simulink model "Privod"  (R2023a)
settings: Solver=ode15s  StartTime=0.0  StopTime=4  RelTol=1e-3
undefined symbols (not defined in the file): a, ak0, ak1, ap0, ap1, bk0, bk1, bp0, bp1, c, F1, F2, G, G1, G2, i, J, k1, k2, Kc, Ki, kip, Kk, km, kpd, kpid, kv, T
settings Model: Creator=manui  LastModifiedBy=manui

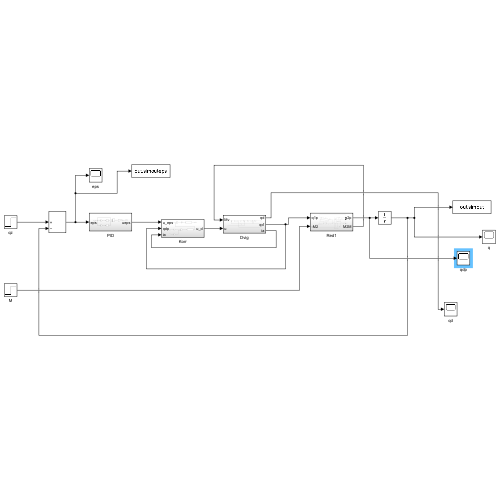
[thumbnail: Simulink's stored preview of the top-level diagram]
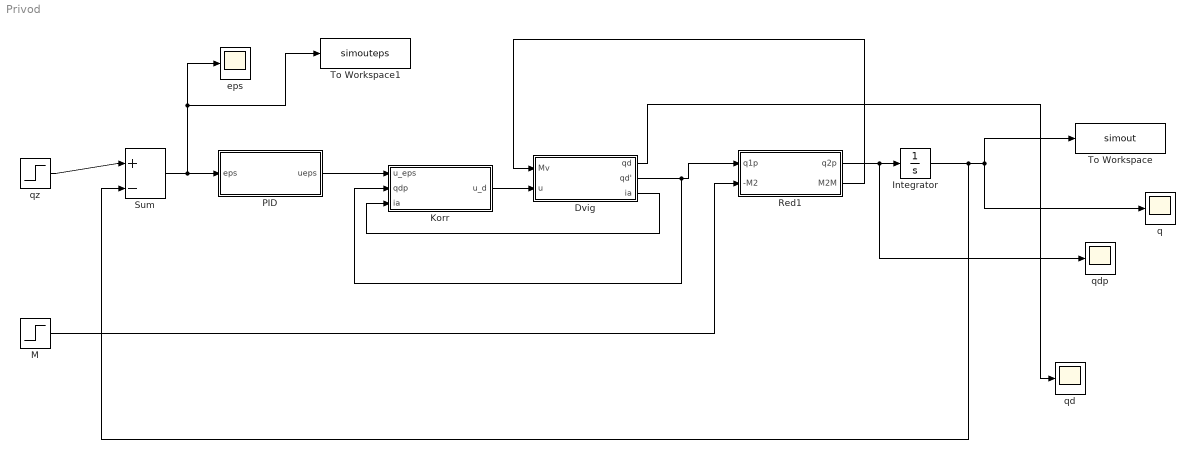
== system Privod ==
  Dvig : Subsystem
  Integrator : Integrator
  Korr : Subsystem
  M : Step  Time=0  After=0  SampleTime=0
  PID : Subsystem
  Red1 : Subsystem
  Sum : Sum  Inputs=|+-
  To Workspace : ToWorkspace  VariableName=simout  SaveFormat=Timeseries  SampleTime=-1
  To Workspace1 : ToWorkspace  VariableName=simouteps  SaveFormat=Timeseries  SampleTime=-1
  eps : Scope
  q : Scope
  qd : Scope
  qdp : Scope
  qz : Step  Time=0  After=0.1  SampleTime=0
  wires:
  qz/1 -> Sum/1
  Sum/1 -> To Workspace1/1, eps/1, PID/1(eps)
  PID/1(ueps) -> Korr/1(u_eps)
  Korr/1(u_d) -> Dvig/2(u)
  Dvig/3(ia) -> Korr/3(ia)
  Dvig/2(qd') -> Korr/2(qdp), Red1/1(q1p)
  M/1 -> Red1/2(-M2)
  Dvig/1(qd) -> qd/1
  Red1/2(M2M) -> Dvig/1(Mv)
  Red1/1(q2p) -> qdp/1, Integrator/1
  Integrator/1 -> Sum/2, To Workspace/1, q/1

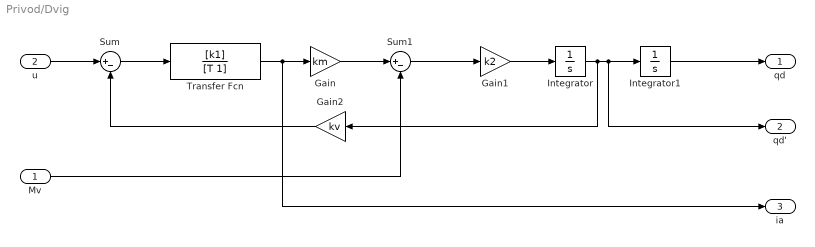
== system Privod/Dvig ==
  Mv : Inport
  u : Inport  Port=2
  Gain : Gain  Gain=km
  Gain1 : Gain  Gain=k2
  Gain2 : Gain  Gain=kv
  Integrator : Integrator
  Integrator1 : Integrator
  Sum : Sum  Inputs=|+-
  Sum1 : Sum  Inputs=|+-
  Transfer Fcn : TransferFcn  Numerator=[k1]  Denominator=[T 1]
  qd : Outport
  qd' : Outport  Port=2
  ia : Outport  Port=3
  wires:
  u/1 -> Sum/1
  Sum/1 -> Transfer Fcn/1
  Transfer Fcn/1 -> ia/1, Gain/1
  Gain/1 -> Sum1/1
  Mv/1 -> Sum1/2
  Sum1/1 -> Gain1/1
  Gain1/1 -> Integrator/1
  Integrator/1 -> Gain2/1, qd'/1, Integrator1/1
  Integrator1/1 -> qd/1
  Gain2/1 -> Sum/2

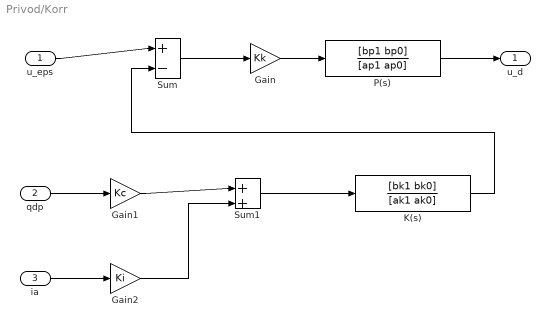
== system Privod/Korr ==
  u_eps : Inport
  qdp : Inport  Port=2
  ia : Inport  Port=3
  Gain : Gain  Gain=Kk
  Gain1 : Gain  Gain=Kc
  Gain2 : Gain  Gain=Ki
  K(s) : TransferFcn  Numerator=[bk1 bk0]  Denominator=[ak1 ak0]
  P(s) : TransferFcn  Numerator=[bp1 bp0]  Denominator=[ap1 ap0]
  Sum : Sum  Inputs=|+-
  Sum1 : Sum  Inputs=|++
  u_d : Outport
  wires:
  Sum/1 -> Gain/1
  u_eps/1 -> Sum/1
  Gain/1 -> P(s)/1
  P(s)/1 -> u_d/1
  qdp/1 -> Gain1/1
  Gain1/1 -> Sum1/1
  Sum1/1 -> K(s)/1
  Gain2/1 -> Sum1/2
  ia/1 -> Gain2/1
  K(s)/1 -> Sum/2

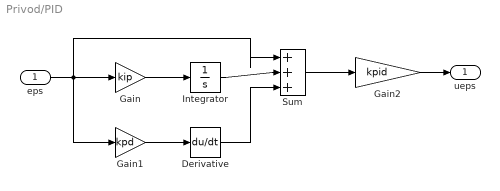
== system Privod/PID ==
  eps : Inport
  Derivative : Derivative
  Gain : Gain  Gain=kip
  Gain1 : Gain  Gain=kpd
  Gain2 : Gain  Gain=kpid
  Integrator : Integrator
  Sum : Sum  Inputs=|+++
  ueps : Outport
  wires:
  eps/1 -> Gain1/1, Sum/1, Gain/1
  Gain/1 -> Integrator/1
  Integrator/1 -> Sum/2
  Gain1/1 -> Derivative/1
  Derivative/1 -> Sum/3
  Sum/1 -> Gain2/1
  Gain2/1 -> ueps/1

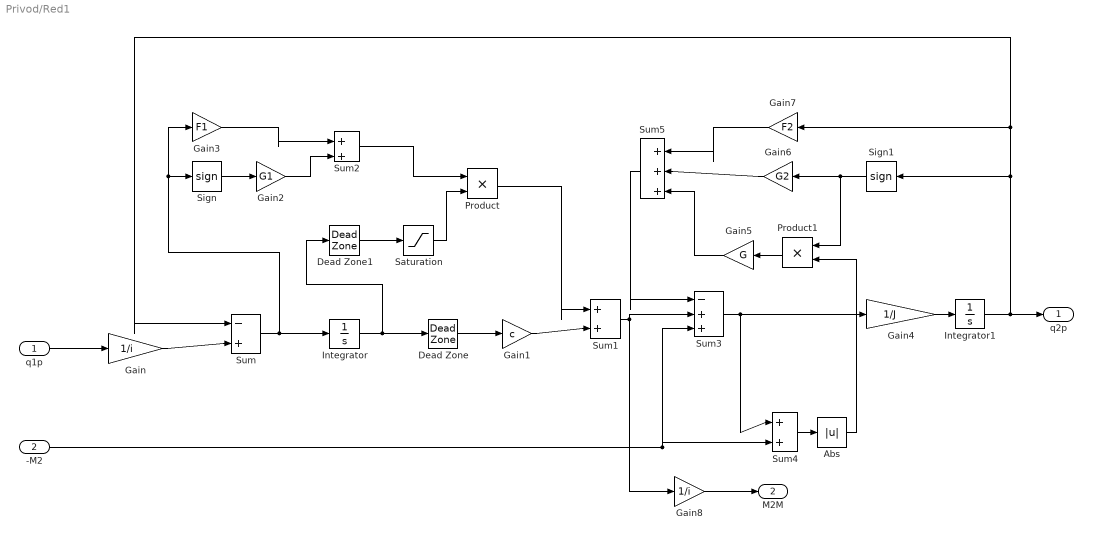
== system Privod/Red1 ==
  q1p : Inport
  -M2 : Inport  Port=2
  Abs : Abs  SaturateOnIntegerOverflow=off
  Dead Zone : DeadZone  LowerValue=-a  UpperValue=a
  Dead Zone1 : DeadZone  LowerValue=-a  UpperValue=a
  Gain : Gain  Gain=1/i
  Gain1 : Gain  Gain=c
  Gain2 : Gain  Gain=G1
  Gain3 : Gain  Gain=F1
  Gain4 : Gain  Gain=1/J
  Gain5 : Gain  Gain=G
  Gain6 : Gain  Gain=G2
  Gain7 : Gain  Gain=F2
  Gain8 : Gain  Gain=1/i
  Integrator : Integrator
  Integrator1 : Integrator
  Product : Product
  Product1 : Product
  Saturation : Saturate  UpperLimit=a  LowerLimit=-a
  Sign : Signum
  Sign1 : Signum
  Sum : Sum  Inputs=|-+
  Sum1 : Sum  Inputs=|++
  Sum2 : Sum  Inputs=|++
  Sum3 : Sum  Inputs=|-++
  Sum4 : Sum  Inputs=|++
  Sum5 : Sum  Inputs=|+++
  q2p : Outport
  M2M : Outport  Port=2
  wires:
  q1p/1 -> Gain/1
  Gain/1 -> Sum/2
  Sum/1 -> Sign/1, Gain3/1, Integrator/1
  Integrator/1 -> Dead Zone1/1, Dead Zone/1
  Dead Zone/1 -> Gain1/1
  Gain1/1 -> Sum1/2
  Product/1 -> Sum1/1
  Saturation/1 -> Product/2
  Dead Zone1/1 -> Saturation/1
  Gain2/1 -> Sum2/2
  Sum2/1 -> Product/1
  Gain3/1 -> Sum2/1
  Sign/1 -> Gain2/1
  Sum1/1 -> Gain8/1, Sum3/2
  -M2/1 -> Sum3/3, Sum4/2
  Gain4/1 -> Integrator1/1
  Integrator1/1 -> Sum/1, Gain7/1, Sign1/1, q2p/1
  Sum3/1 -> Sum4/1, Gain4/1
  Sum4/1 -> Abs/1
  Abs/1 -> Product1/2
  Product1/1 -> Gain5/1
  Gain5/1 -> Sum5/3
  Gain6/1 -> Sum5/2
  Sign1/1 -> Product1/1, Gain6/1
  Gain7/1 -> Sum5/1
  Gain8/1 -> M2M/1
  Sum5/1 -> Sum3/1
